simulink model "sedemo_ethernet"  (Simulink 7.5)
settings: Solver=VariableStepDiscrete  StartTime=0.0  StopTime=10.0  MaxStep=inf  RelTol=1e-3
PreLoadFcn:
  | MACInputSize = 25;
  | warning('off','MATLAB:divideByZero');
undefined symbols (not defined in the file or in its folder): des_subsystemblock, des_subsysteminport, des_subsystemoutport, des_subsystemsupportblock
libraries: simeventsrouting1 x30, simeventstranslate1 x26, simeventsattributes2 x16, simeventssink1 x13, simeventsserver1 x13, simeventsgenerators1 x11, simeventssignalmanage1 x9, simeventsgates1 x6, simeventsqueue1 x3, simeventsinfo x1
(part 5 of 5)

== system sedemo_ethernet/MAC Controller (C)/CSMA/CD/Discrete Event Subsystem (Carrier Sensing)/__fcn_ss__ ==
  l_status : Inport  LoadFcn=des_subsysteminport(gcb, 'load');  InitFcn=des_subsysteminport(gcb, 'init');  StartFcn=des_subsysteminport(gcb, 'start');  StopFcn=des_subsysteminport(gcb, 'stop');  OutDataType=sfix(16)  OutScaling=2^0  mask(Discrete Event Inport){PermitSubsystemEvents=on, TypeOfEvent=Sample time hit, SignalEdgeOption=Rising, SpecifyEventPriority=off, PrioritySubsystemEvent=20}
      mask prompts: PermitSubsystemEvents "Execute subsystem upon signal-based events"; TypeOfEvent "Type of signal-based event:"; SignalEdgeOption "Type of change in signal value:"; SpecifyEventPriority "Specify event priority for executing subsystem"; PrioritySubsystemEvent "Subsystem execution event priority:"
      mask help: Input port for a Discrete Event Subsystem block. This block can conditionally execute the subsystem upon signal-based events that meet specified criteria.
      mask init:
      | des_subsystemmask(gcb, 'init','apply')
      settings: CopyFcn=des_subsysteminport(gcb, 'copy');  DeleteFcn=des_subsysteminport(gcb, 'delete');  UndoDeleteFcn=des_subsysteminport(gcb, 'undodelete');  ModelCloseFcn=des_subsysteminport(gcb, 'modelclose');  PreSaveFcn=des_subsysteminport(gcb, 'presave');  NameChangeFcn=des_subsysteminport(gcb, 'namechange');  ParentCloseFcn=des_subsysteminport(gcb, 'parentclose');
      mask Help: helpview(simeventsbhelp);
      mask StyleString: checkbox,popup(Change in signal|Trigger|Sample time hit),popup(Rising|Falling|Either),checkbox,edit
      mask CallbackString: des_subsystemmask(gcb, 'cbPermitSubsystemEvents', 'noapply');|des_subsystemmask(gcb,'cbTypeOfEvent','noapply');||des_subsystemmask(gcb, 'cbSpecifyEventPriority', 'noapply');|
  Subsystem Configuration : TriggerPort  TriggerType=function-call
      settings: CopyFcn=des_subsystemconfigblock(gcb, 'copy');  DeleteFcn=des_subsystemconfigblock(gcb, 'delete');  UndoDeleteFcn=des_subsystemconfigblock(gcb, 'undodelete');
      mask Type: Subsystem Configuration
      mask Description: Configuration for a Discrete Event Subsystem block. Every discrete event subsystem window must contain exactly one copy of this configuration block. Do not delete this block.
      mask Help: helpview(simeventsbhelp);
      mask Display: disp('Do Not Delete');
  Constant : Constant  Value=1+eps  OutDataType=sfix(16)  OutScaling=2^0
  Constant1 : Constant  OutDataType=sfix(16)  OutScaling=2^0
  Sum : Sum  Inputs=|-+  OutDataType=sfix(16)  OutScaling=2^0
  Sum1 : Sum  Inputs=|+-  OutDataType=sfix(16)  OutScaling=2^0
  l_ready : Outport  LoadFcn=des_subsystemoutport(gcb, 'load');  InitFcn=des_subsystemoutport(gcb, 'init');  StartFcn=des_subsystemoutport(gcb, 'start');  StopFcn=des_subsystemoutport(gcb, 'stop');  OutDataType=sfix(16)  OutScaling=2^0  InitialOutput=1  mask(Discrete Event Outport){InitOutput=1}
      mask prompts: InitOutput "Initial output:"
      mask help: Provide an output port for a Discrete Event Subsystem block.
      settings: CopyFcn=des_subsystemoutport(gcb, 'copy');  DeleteFcn=des_subsystemoutport(gcb, 'delete');  UndoDeleteFcn=des_subsystemoutport(gcb, 'undodelete');  ModelCloseFcn=des_subsystemoutport(gcb, 'modelclose');  PreSaveFcn=des_subsystemoutport(gcb, 'presave');  NameChangeFcn=des_subsystemoutport(gcb, 'namechange');  ParentCloseFcn=des_subsystemoutport(gcb, 'parentclose');
      mask Help: helpview(simeventsbhelp);
      mask CallbackString: set_param(gcb,'InitialOutput',get_param(gcb,'InitOutput'));
  collision : Outport  LoadFcn=des_subsystemoutport(gcb, 'load');  InitFcn=des_subsystemoutport(gcb, 'init');  StartFcn=des_subsystemoutport(gcb, 'start');  StopFcn=des_subsystemoutport(gcb, 'stop');  Port=2  OutDataType=sfix(16)  OutScaling=2^0  InitialOutput=0  mask(Discrete Event Outport){InitOutput=0}
      mask prompts: InitOutput "Initial output:"
      mask help: Provide an output port for a Discrete Event Subsystem block.
      settings: CopyFcn=des_subsystemoutport(gcb, 'copy');  DeleteFcn=des_subsystemoutport(gcb, 'delete');  UndoDeleteFcn=des_subsystemoutport(gcb, 'undodelete');  ModelCloseFcn=des_subsystemoutport(gcb, 'modelclose');  PreSaveFcn=des_subsystemoutport(gcb, 'presave');  NameChangeFcn=des_subsystemoutport(gcb, 'namechange');  ParentCloseFcn=des_subsystemoutport(gcb, 'parentclose');
      mask Help: helpview(simeventsbhelp);
      mask CallbackString: set_param(gcb,'InitialOutput',get_param(gcb,'InitOutput'));
  wires:
  Sum1/1 -> l_ready/1
  Constant1/1 -> Sum1/1
  Sum/1 -> collision/1
  l_status/1 -> Sum1/2, Sum/2
  Constant/1 -> Sum/1

== system sedemo_ethernet/MAC Controller (C)/Transmission Buffer Controller/Transmission Buffer Controller/AAA___ ==

== system sedemo_ethernet/MAC Controller (C)/Transmission Buffer Controller/Transmission Buffer Controller/__fcn_ss__ ==
  #tx : Inport  LoadFcn=des_subsysteminport(gcb, 'load');  InitFcn=des_subsysteminport(gcb, 'init');  StartFcn=des_subsysteminport(gcb, 'start');  StopFcn=des_subsysteminport(gcb, 'stop');  OutDataType=sfix(16)  OutScaling=2^0  mask(Discrete Event Inport){PermitSubsystemEvents=on, TypeOfEvent=Sample time hit, SignalEdgeOption=Rising, SpecifyEventPriority=off, PrioritySubsystemEvent=20}
      mask prompts: PermitSubsystemEvents "Execute subsystem upon signal-based events"; TypeOfEvent "Type of signal-based event:"; SignalEdgeOption "Type of change in signal value:"; SpecifyEventPriority "Specify event priority for executing subsystem"; PrioritySubsystemEvent "Subsystem execution event priority:"
      mask help: Input port for a Discrete Event Subsystem block. This block can conditionally execute the subsystem upon signal-based events that meet specified criteria.
      mask init:
      | des_subsystemmask(gcb, 'init','apply')
      settings: CopyFcn=des_subsysteminport(gcb, 'copy');  DeleteFcn=des_subsysteminport(gcb, 'delete');  UndoDeleteFcn=des_subsysteminport(gcb, 'undodelete');  ModelCloseFcn=des_subsysteminport(gcb, 'modelclose');  PreSaveFcn=des_subsysteminport(gcb, 'presave');  NameChangeFcn=des_subsysteminport(gcb, 'namechange');  ParentCloseFcn=des_subsysteminport(gcb, 'parentclose');
      mask Help: helpview(simeventsbhelp);
      mask StyleString: checkbox,popup(Change in signal|Trigger|Sample time hit),popup(Rising|Falling|Either),checkbox,edit
      mask CallbackString: des_subsystemmask(gcb, 'cbPermitSubsystemEvents', 'noapply');|des_subsystemmask(gcb,'cbTypeOfEvent','noapply');||des_subsystemmask(gcb, 'cbSpecifyEventPriority', 'noapply');|
  #success : Inport  LoadFcn=des_subsysteminport(gcb, 'load');  InitFcn=des_subsysteminport(gcb, 'init');  StartFcn=des_subsysteminport(gcb, 'start');  StopFcn=des_subsysteminport(gcb, 'stop');  Port=2  OutDataType=sfix(16)  OutScaling=2^0  mask(Discrete Event Inport){PermitSubsystemEvents=on, TypeOfEvent=Sample time hit, SignalEdgeOption=Rising, SpecifyEventPriority=off, PrioritySubsystemEvent=20}
      mask prompts: PermitSubsystemEvents "Execute subsystem upon signal-based events"; TypeOfEvent "Type of signal-based event:"; SignalEdgeOption "Type of change in signal value:"; SpecifyEventPriority "Specify event priority for executing subsystem"; PrioritySubsystemEvent "Subsystem execution event priority:"
      mask help: Input port for a Discrete Event Subsystem block. This block can conditionally execute the subsystem upon signal-based events that meet specified criteria.
      mask init:
      | des_subsystemmask(gcb, 'init','apply')
      settings: CopyFcn=des_subsysteminport(gcb, 'copy');  DeleteFcn=des_subsysteminport(gcb, 'delete');  UndoDeleteFcn=des_subsysteminport(gcb, 'undodelete');  ModelCloseFcn=des_subsysteminport(gcb, 'modelclose');  PreSaveFcn=des_subsysteminport(gcb, 'presave');  NameChangeFcn=des_subsysteminport(gcb, 'namechange');  ParentCloseFcn=des_subsysteminport(gcb, 'parentclose');
      mask Help: helpview(simeventsbhelp);
      mask StyleString: checkbox,popup(Change in signal|Trigger|Sample time hit),popup(Rising|Falling|Either),checkbox,edit
      mask CallbackString: des_subsystemmask(gcb, 'cbPermitSubsystemEvents', 'noapply');|des_subsystemmask(gcb,'cbTypeOfEvent','noapply');||des_subsystemmask(gcb, 'cbSpecifyEventPriority', 'noapply');|
  #failure : Inport  LoadFcn=des_subsysteminport(gcb, 'load');  InitFcn=des_subsysteminport(gcb, 'init');  StartFcn=des_subsysteminport(gcb, 'start');  StopFcn=des_subsysteminport(gcb, 'stop');  Port=3  OutDataType=sfix(16)  OutScaling=2^0  mask(Discrete Event Inport){PermitSubsystemEvents=on, TypeOfEvent=Sample time hit, SignalEdgeOption=Rising, SpecifyEventPriority=off, PrioritySubsystemEvent=20}
      mask prompts: PermitSubsystemEvents "Execute subsystem upon signal-based events"; TypeOfEvent "Type of signal-based event:"; SignalEdgeOption "Type of change in signal value:"; SpecifyEventPriority "Specify event priority for executing subsystem"; PrioritySubsystemEvent "Subsystem execution event priority:"
      mask help: Input port for a Discrete Event Subsystem block. This block can conditionally execute the subsystem upon signal-based events that meet specified criteria.
      mask init:
      | des_subsystemmask(gcb, 'init','apply')
      settings: CopyFcn=des_subsysteminport(gcb, 'copy');  DeleteFcn=des_subsysteminport(gcb, 'delete');  UndoDeleteFcn=des_subsysteminport(gcb, 'undodelete');  ModelCloseFcn=des_subsysteminport(gcb, 'modelclose');  PreSaveFcn=des_subsysteminport(gcb, 'presave');  NameChangeFcn=des_subsysteminport(gcb, 'namechange');  ParentCloseFcn=des_subsysteminport(gcb, 'parentclose');
      mask Help: helpview(simeventsbhelp);
      mask StyleString: checkbox,popup(Change in signal|Trigger|Sample time hit),popup(Rising|Falling|Either),checkbox,edit
      mask CallbackString: des_subsystemmask(gcb, 'cbPermitSubsystemEvents', 'noapply');|des_subsystemmask(gcb,'cbTypeOfEvent','noapply');||des_subsystemmask(gcb, 'cbSpecifyEventPriority', 'noapply');|
  Subsystem Configuration : TriggerPort  TriggerType=function-call
      settings: CopyFcn=des_subsystemconfigblock(gcb, 'copy');  DeleteFcn=des_subsystemconfigblock(gcb, 'delete');  UndoDeleteFcn=des_subsystemconfigblock(gcb, 'undodelete');
      mask Type: Subsystem Configuration
      mask Description: Configuration for a Discrete Event Subsystem block. Every discrete event subsystem window must contain exactly one copy of this configuration block. Do not delete this block.
      mask Help: helpview(simeventsbhelp);
      mask Display: disp('Do Not Delete');
  Constant : Constant  OutDataType=sfix(16)  OutScaling=2^0
  Subtract : Sum  Inputs=+-++  OutDataType=sfix(16)  OutScaling=2^-10
  state : Outport  LoadFcn=des_subsystemoutport(gcb, 'load');  InitFcn=des_subsystemoutport(gcb, 'init');  StartFcn=des_subsystemoutport(gcb, 'start');  StopFcn=des_subsystemoutport(gcb, 'stop');  OutDataType=sfix(16)  OutScaling=2^0  mask(Discrete Event Outport){InitOutput=[]}
      mask prompts: InitOutput "Initial output:"
      mask help: Provide an output port for a Discrete Event Subsystem block.
      settings: CopyFcn=des_subsystemoutport(gcb, 'copy');  DeleteFcn=des_subsystemoutport(gcb, 'delete');  UndoDeleteFcn=des_subsystemoutport(gcb, 'undodelete');  ModelCloseFcn=des_subsystemoutport(gcb, 'modelclose');  PreSaveFcn=des_subsystemoutport(gcb, 'presave');  NameChangeFcn=des_subsystemoutport(gcb, 'namechange');  ParentCloseFcn=des_subsystemoutport(gcb, 'parentclose');
      mask Help: helpview(simeventsbhelp);
      mask CallbackString: set_param(gcb,'InitialOutput',get_param(gcb,'InitOutput'));
  wires:
  Subtract/1 -> state/1
  Constant/1 -> Subtract/1
  #tx/1 -> Subtract/2
  #success/1 -> Subtract/3
  #failure/1 -> Subtract/4

== stateflow chart MAC Controller (C)/Backoff Controller/__fcn_ss__/Chart ==
  settings: initializeOutput=1
  state PacketSource [parallel]
    settings: executionOrder=1
    state Transmitting
      state TxOK
        route=2;
        newColliNum=numCollision;
        bckoffTime=0;
      state Collision
        state TxRetry
          route=4;
          newColliNum = numCollision + 1;
          total++;
          bckoffTime=Backoff(newColliNum);
        state TxFail
          route=3;
          newColliNum = numCollision + 1;
          total++;
          bckoffTime=0;
          num++;
        (junction 19) -> TxRetry [order 1] : [numCollision<15]
        (default) -> (junction 19)
        (junction 19) -> TxFail [order 2]
      (junction 18) -> Collision [order 2]
      (default) -> (junction 18)
      (junction 18) -> TxOK [order 1] : [!collision]
    state Receiving
      state RxOK
        route=1;
        newColliNum=numCollision;
        bckoffTime=0;
      state RxFail
        route=3;
        newColliNum=numCollision+1;
        bckoffTime=0;
      (default) -> (junction 17)
      (junction 17) -> RxOK [order 1] : [!collision]
      (junction 17) -> RxFail [order 2]
    (default) -> (junction 16) : {InitRand()}
    (junction 16) -> Transmitting [order 1] : [srcAddress==myAddress]
    (junction 16) -> Receiving [order 2]
    PacketSource -> (junction 16)
  state UpdateStats [parallel]
    settings: executionOrder=2
    state Update
      failure=num;
      sum=total;
    Update -> Update
  data: t function_output double; u function_input double; srcAddress input double; myAddress input double; numCollision input double; sum output double; failure output double; route output double; newColliNum output double; bckoffTime output double; num local double =0; total local double =0; collision input double
  function t = Backoff(u):
    | function t = Backoff(u)
    | t = floor(rand*(2^min([u,10])))*5.12e-5;
  function InitRand:
    | function InitRand
    | rand('seed',srcAddress);

== matlab function MAC Controller (B)/Compute channel utilization/__fcn_ss__/Embedded MATLAB Function ==
  data: cur_T input double; cur_st input double; util output double
function util = utilization(cur_T, cur_st)
%UTILIZATION Compute fraction of time that a signal is positive.
%   UTIL = UTILIZATION(CUR_T,CUR_ST) computes the fraction of
%   time that the input CUR_ST is positive, where CUR_T is the
%   current simulation time.

persistent acc_sum last_T last_st;

% Initialize persistent variables in the first iteration.
if isempty(last_T)
   acc_sum = 0;
   last_T = 0;
   last_st = 0;
end

% Keep running total of the duration that the signal is positive.
if(last_st>0)
    acc_sum = acc_sum + (cur_T-last_T);
end

% Update the other persistent variables.
last_T = cur_T;
last_st = cur_st;

% Compute ratio.
util = acc_sum / cur_T;

== stateflow chart MAC Controller (B)/Backoff Controller/__fcn_ss__/Chart ==
  settings: initializeOutput=1
  state PacketSource [parallel]
    settings: executionOrder=1
    state Transmitting
      state TxOK
        route=2;
        newColliNum=numCollision;
        bckoffTime=0;
      state Collision
        state TxRetry
          route=4;
          newColliNum = numCollision + 1;
          total++;
          bckoffTime=Backoff(newColliNum);
        state TxFail
          route=3;
          newColliNum = numCollision + 1;
          total++;
          bckoffTime=0;
          num++;
        (junction 73) -> TxRetry [order 1] : [numCollision<15]
        (default) -> (junction 73)
        (junction 73) -> TxFail [order 2]
      (junction 72) -> Collision [order 2]
      (default) -> (junction 72)
      (junction 72) -> TxOK [order 1] : [!collision]
    state Receiving
      state RxOK
        route=1;
        newColliNum=numCollision;
        bckoffTime=0;
      state RxFail
        route=3;
        newColliNum=numCollision+1;
        bckoffTime=0;
      (default) -> (junction 71)
      (junction 71) -> RxOK [order 1] : [!collision]
      (junction 71) -> RxFail [order 2]
    (default) -> (junction 70) : {InitRand()}
    (junction 70) -> Transmitting [order 1] : [srcAddress==myAddress]
    (junction 70) -> Receiving [order 2]
    PacketSource -> (junction 70)
  state UpdateStats [parallel]
    settings: executionOrder=2
    state Update
      failure=num;
      sum=total;
    Update -> Update
  data: t function_output double; u function_input double; srcAddress input double; myAddress input double; numCollision input double; sum output double; failure output double; route output double; newColliNum output double; bckoffTime output double; num local double =0; total local double =0; collision input double
  function t = Backoff(u):
    | function t = Backoff(u)
    | t = floor(rand*(2^min([u,10])))*5.12e-5;
  function InitRand:
    | function InitRand
    | rand('seed',srcAddress);

== stateflow chart MAC Controller (A)/Backoff Controller/__fcn_ss__/Chart ==
  settings: initializeOutput=1
  state PacketSource [parallel]
    settings: executionOrder=1
    state Transmitting
      state TxOK
        route=2;
        newColliNum=numCollision;
        bckoffTime=0;
      state Collision
        state TxRetry
          route=4;
          newColliNum = numCollision + 1;
          total++;
          bckoffTime=Backoff(newColliNum);
        state TxFail
          route=3;
          newColliNum = numCollision + 1;
          total++;
          bckoffTime=0;
          num++;
        (junction 119) -> TxRetry [order 1] : [numCollision<15]
        (default) -> (junction 119)
        (junction 119) -> TxFail [order 2]
      (junction 118) -> Collision [order 2]
      (default) -> (junction 118)
      (junction 118) -> TxOK [order 1] : [!collision]
    state Receiving
      state RxOK
        route=1;
        newColliNum=numCollision;
        bckoffTime=0;
      state RxFail
        route=3;
        newColliNum=numCollision+1;
        bckoffTime=0;
      (default) -> (junction 117)
      (junction 117) -> RxOK [order 1] : [!collision]
      (junction 117) -> RxFail [order 2]
    (default) -> (junction 116) : {InitRand()}
    (junction 116) -> Transmitting [order 1] : [srcAddress==myAddress]
    (junction 116) -> Receiving [order 2]
    PacketSource -> (junction 116)
  state UpdateStats [parallel]
    settings: executionOrder=2
    state Update
      failure=num;
      sum=total;
    Update -> Update
  data: t function_output double; u function_input double; srcAddress input double; myAddress input double; numCollision input double; sum output double; failure output double; route output double; newColliNum output double; bckoffTime output double; num local double =0; total local double =0; collision input double
  function t = Backoff(u):
    | function t = Backoff(u)
    | t = floor(rand*(2^min([u,10])))*5.12e-5;
  function InitRand:
    | function InitRand
    | rand('seed',srcAddress);

== matlab function MAC Controller (B)/Compute Tx throughput/__fcn_ss__/Embedded MATLAB Function ==
  data: cur_T input double; pck_size input double; rate output double
function rate = throughput(cur_T, pck_size)
% THROUGHPUT Compute the rate at which the computer sends data 
% INPUT:
%     cur_T     -- Current simulation time
%     pck_size  -- Size, in bits, of the packet that is successfully
%                  transmitted.
% OUTPUT:
%     rate      -- Current throughput of the computer (in kbps)

persistent acc_sum;

% Initialize persistent variables in the first iteration.
if isempty(acc_sum)
   acc_sum = 0;
end

% Update the throughput of current computer.
acc_sum = acc_sum + pck_size;
rate = acc_sum / (1000*cur_T);
